simulink model "complex_UIO_alternative_proj_2021_02_16"  (R2019b)
settings: Solver=FixedStepAuto  StartTime=0.0  StopTime=60  FixedStep=0.1  RelTol=1e-3
values from neighbouring files (symbols this model uses):
  Ac = [real(A) -imag(A);imag(A) real(A)]    [DAC_UIO_Comp.m]    (also in LinearND_QUANTUM_2020_11_14_2.m = [realA -imagA;imagA realA]; UIO_alternative_2021_01_26.m; UIO_alternative_PAPER_2021_02_17.m = Abar(2:3,2:3); UIO_alternative_PAPER_2021_03_01.m = Abar(2:3,2:3))
  Amc = [real(Am) -imag(Am);imag(Am) real(Am)]    [DAC_UIO_Comp.m]    (also in UIO_alternative_2021_01_26.m)
  Bc = [real(B) -imag(B);imag(B) real(B)]    [DAC_UIO_Comp.m]    (also in UIO_alternative_2021_01_26.m; UIO_alternative_PAPER_2021_02_17.m = Bbar(2:3,:); UIO_alternative_PAPER_2021_03_01.m = Bbar(2:3,:))
  C = double(subs(C_sym,{ep},{0.1}))    [DAC_UIO_Comp.m]    (also in UIO_adaptive_example.m = [1 0 0 0 0;0 0 0 1 0; 0 0 0 0 1]; UIO_adaptive_example_2.m = [1 0 0 0;0 1 0 0]; UIO_adaptive_example_EEG_Balas_2ch.m = [1, epsilon]; UIO_adaptive_example_alternative_EEG_ch6.m = ss_c.C)
  Fu = mats    [UIO_adaptive_example_alternative_EEG_ch6.m]    (also in UIO_alternative_2021_01_26.m = [0 1 ;-25 0]; UIO_alternative_PAPER_2021_02_17.m = [0,0,0,0, 0;0 0 1 0 0;0 -25 0 0 0;0 0 0 0 1;0 0 0 -144 0]; UIO_alternative_PAPER_2021_03_01.m = [0 1 0 0;-25 0 0 0;0 0 0 1;0 0 -144 0]; UIO_alternative_PAPER_2021_03_02.m = [0 1 0 0;-25 0 0 0;0 0 0 1;0 0 -144 0])
  g1 = 4+2j    [DAC_UIO_Comp.m]    (also in UIO_adaptive_example_EEG_Balas_2ch.m = 4; UIO_alternative_2021_01_26.m = 2+1j; UIO_alternative_PAPER_2021_02_17.m = 2; UIO_alternative_PAPER_2021_03_01.m = 2)
  g2 = 0    [DAC_UIO_Comp.m]    (also in UIO_adaptive_example_EEG_Balas_2ch.m = -0.3; UIO_alternative_2021_01_26.m; UIO_alternative_PAPER_2021_02_17.m = 1; UIO_alternative_PAPER_2021_03_01.m)
  g3 = 0    [DAC_UIO_Comp.m]    (also in UIO_adaptive_example_EEG_Balas_2ch.m = 0.1; UIO_alternative_2021_01_26.m; UIO_alternative_PAPER_2021_02_17.m = -3; UIO_alternative_PAPER_2021_03_01.m)
  gamma_e = 1    [DAC_UIO_Comp.m]    (also in UIO_adaptive_example_EEG_Balas_2ch.m; UIO_adaptive_example_alternative_EEG_ch6.m = .0001*ones(length(Am),1); UIO_alternative_2021_01_26.m = 0.001; UIO_alternative_PAPER_2021_02_17.m = 0.0001)
  K_u = ones(size(Fu,1),1)    [UIO_adaptive_example_alternative_EEG_ch6.m]    (also in UIO_alternative_2021_01_26.m = [0.215;ku]; UIO_alternative_PAPER_2021_02_17.m = [2;10;-1.6;10]; UIO_alternative_PAPER_2021_03_01.m = -[K_cvx(3:end,:)]; UIO_alternative_PAPER_2021_03_02.m)
  Theta = [real(Theta_cust);imag(Theta_cust)]    [LinearND_QUANTUM_2020_11_14_2.m]    (also in UIO_adaptive_example_alternative_EEG_ch6.m = ones(1,size(Fu,1)); UIO_alternative_2021_01_26.m = [1,1]; UIO_alternative_PAPER_2021_02_17.m = [1,1,1,1,1]; UIO_alternative_PAPER_2021_03_01.m = [1,1,1,1])
settings Model: Creator=Tris  LastModifiedBy=Tris

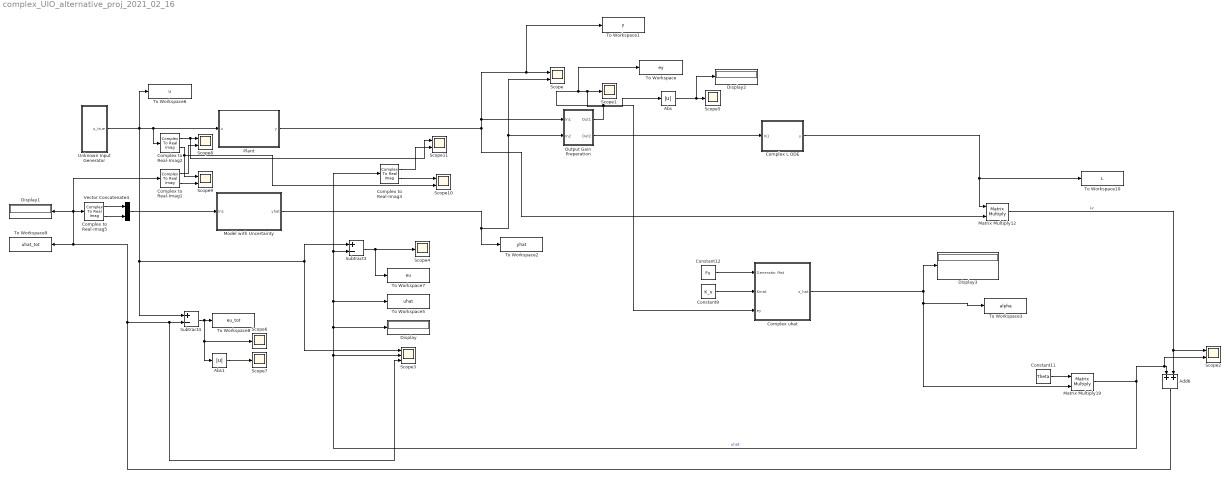
== system complex_UIO_alternative_proj_2021_02_16 ==
  Abs : Abs
  Abs1 : Abs
  Add6 : Sum
  Complex L ODE : Subsystem
  Complex to Real-Imag{1..3,5} (4 alike) : ComplexToRealImag
  "Complex uhat " : Subsystem
  Constant11 : Constant  Value=Theta  VectorParams1D=off
  Constant12 : Constant  Value=Fu
  Constant9 : Constant  Value=K_u  VectorParams1D=off
  Display{,1..3} (4 alike) : Display
  Matrix Multiply12 : Product  Multiplication=Matrix(*)
  Matrix Multiply19 : Product  Multiplication=Matrix(*)
  Model with Uncertainty : Subsystem
  Output Gain Preperation : Subsystem
  Plant : Subsystem
  Scope{,2,8..11} (6 alike) : Scope  NumInputPorts=2
  Scope{1,4..7} (5 alike) : Scope
  Scope3 : Scope  NumInputPorts=3
  Subtract3 : Sum  Inputs=+-
  Subtract4 : Sum  Inputs=+-
  To Workspace : ToWorkspace  VariableName=ey  SaveFormat=Timeseries  SampleTime=-1
  To Workspace1 : ToWorkspace  VariableName=y  SaveFormat=Timeseries  SampleTime=-1
  To Workspace10 : ToWorkspace  VariableName=L  SaveFormat=Timeseries  SampleTime=-1
  To Workspace2 : ToWorkspace  VariableName=yhat  SaveFormat=Timeseries  SampleTime=-1
  To Workspace3 : ToWorkspace  VariableName=alpha  SaveFormat=Timeseries  SampleTime=-1
  To Workspace5 : ToWorkspace  VariableName=uhat  SaveFormat=Timeseries  SampleTime=-1
  To Workspace6 : ToWorkspace  VariableName=u  SaveFormat=Timeseries  SampleTime=-1
  To Workspace7 : ToWorkspace  VariableName=eu  SaveFormat=Timeseries  SampleTime=-1
  To Workspace8 : ToWorkspace  VariableName=eu_tot  SaveFormat=Timeseries  SampleTime=-1
  To Workspace9 : ToWorkspace  VariableName=uhat_tot  SaveFormat=Timeseries  SampleTime=-1
  Unknown Input Generator : Subsystem
  Vector Concatenate4 : Concatenate  Mode=Multidimensional array
  wires:
  Complex to Real-Imag5/2 -> Vector Concatenate4/2
  Complex to Real-Imag5/1 -> Vector Concatenate4/1
  Constant11/1 -> Matrix Multiply19/1
  Matrix Multiply19/1 -> Scope2/2, Add6/1, To Workspace5/1, Complex to Real-Imag3/1, Subtract3/2, Display/1, Scope3/2  "uhat"
  Matrix Multiply12/1 -> Scope2/1, Add6/2  "Ly"
  Add6/1 -> Complex to Real-Imag1/1, Complex to Real-Imag5/1, Display1/1, To Workspace9/1, Scope3/3, Subtract4/2
  Subtract4/1 -> Abs1/1, Scope6/1, To Workspace8/1
  Constant9/1 -> "Complex uhat "/2(Kmat)
  Constant12/1 -> "Complex uhat "/1(Generator Mat)
  "Complex uhat "/1(z_hat) -> To Workspace3/1, Matrix Multiply19/2, Display3/1
  Complex L ODE/1(y) -> To Workspace10/1, Matrix Multiply12/1
  Plant/1(y) -> To Workspace1/1, Scope/1, Output Gain Preperation/1(In1), Matrix Multiply12/2
  Abs/1 -> Display2/1, Scope5/1
  Unknown Input Generator/1(u_true) -> Scope3/1, Subtract3/1, Subtract4/1, To Workspace6/1, Complex to Real-Imag2/1, Plant/1(u)
  Model with Uncertainty/1(yhat) -> To Workspace2/1, Scope/2, Output Gain Preperation/2(In2)
  Vector Concatenate4/1 -> Model with Uncertainty/1(In1)
  Subtract3/1 -> Scope4/1, To Workspace7/1
  Output Gain Preperation/1(Out1) -> To Workspace/1, Abs/1, Scope1/1, "Complex uhat "/3(ey)
  Output Gain Preperation/2(Out2) -> Complex L ODE/1(In1)
  Abs1/1 -> Scope7/1
  Complex to Real-Imag2/1 -> Scope11/1, Scope8/1
  Complex to Real-Imag1/1 -> Scope8/2
  Complex to Real-Imag1/2 -> Scope9/2
  Complex to Real-Imag2/2 -> Scope10/2, Scope9/1
  Complex to Real-Imag3/1 -> Scope11/2
  Complex to Real-Imag3/2 -> Scope10/1

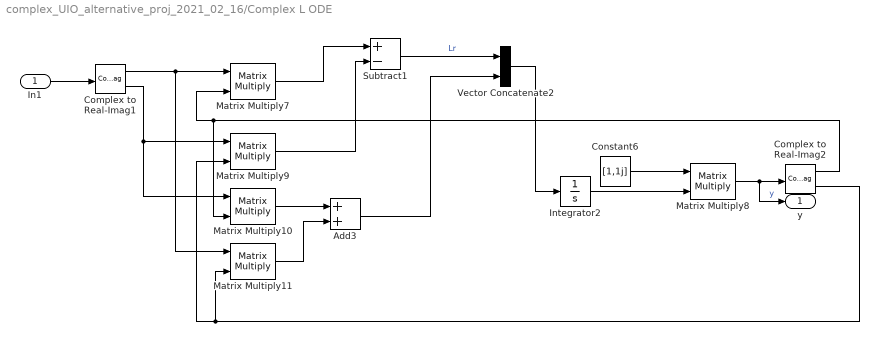
== system complex_UIO_alternative_proj_2021_02_16/Complex L ODE ==
  In1 : Inport
  Add3 : Sum
  Complex to Real-Imag1 : ComplexToRealImag
  Complex to Real-Imag2 : ComplexToRealImag
  Constant6 : Constant  Value=[1,1j]  VectorParams1D=off
  Integrator2 : Integrator  InitialCondition=[1;0.5]
  Matrix Multiply{7..11} (5 alike) : Product  Multiplication=Matrix(*)
  Subtract1 : Sum  Inputs=+-
  Vector Concatenate2 : Concatenate  Mode=Multidimensional array
  y : Outport
  wires:
  Complex to Real-Imag2/1 -> Matrix Multiply7/2, Matrix Multiply10/2
  Matrix Multiply8/1 -> y/1, Complex to Real-Imag2/1  "y"
  Complex to Real-Imag2/2 -> Matrix Multiply11/2, Matrix Multiply9/2
  Subtract1/1 -> Vector Concatenate2/1  "Lr"
  Add3/1 -> Vector Concatenate2/2
  Complex to Real-Imag1/2 -> Matrix Multiply10/1, Matrix Multiply9/1
  Constant6/1 -> Matrix Multiply8/1
  Matrix Multiply10/1 -> Add3/1
  Complex to Real-Imag1/1 -> Matrix Multiply11/1, Matrix Multiply7/1
  Matrix Multiply7/1 -> Subtract1/1
  Integrator2/1 -> Matrix Multiply8/2
  Matrix Multiply9/1 -> Subtract1/2
  Vector Concatenate2/1 -> Integrator2/1
  Matrix Multiply11/1 -> Add3/2
  In1/1 -> Complex to Real-Imag1/1

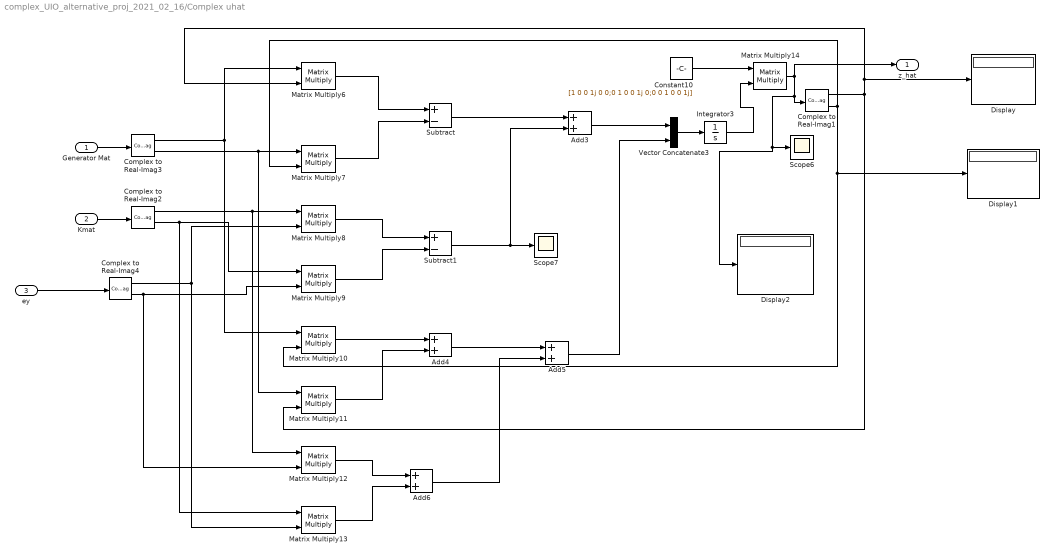
== system complex_UIO_alternative_proj_2021_02_16/Complex uhat  ==
  Generator Mat : Inport
  Kmat : Inport  Port=2
  ey : Inport  Port=3
  Add{3..6} (4 alike) : Sum
  Complex to Real-Imag{1..4} (4 alike) : ComplexToRealImag
  Constant10 : Constant  Value=[1 0 0 1j 0 0;0 1 0 0 1j 0;0 0 1 0 0 1j]  VectorParams1D=off
  Display : Display
  Display1 : Display
  Display2 : Display
  Integrator3 : Integrator  InitialCondition=[2;0;1;0;0;0]  LimitOutput=on
  Matrix Multiply{6..14} (9 alike) : Product  Multiplication=Matrix(*)
  Scope6 : Scope
  Scope7 : Scope
  Subtract : Sum  Inputs=+-
  Subtract1 : Sum  Inputs=+-
  Vector Concatenate3 : Concatenate  Mode=Multidimensional array
  z_hat : Outport
  wires:
  ey/1 -> Complex to Real-Imag4/1
  Matrix Multiply9/1 -> Subtract1/2
  Integrator3/1 -> Matrix Multiply14/2
  Matrix Multiply6/1 -> Subtract/1
  Add5/1 -> Vector Concatenate3/2
  Matrix Multiply14/1 -> Complex to Real-Imag1/1, Scope6/1, Display2/1, z_hat/1
  Matrix Multiply7/1 -> Subtract/2
  Subtract/1 -> Add3/1
  Matrix Multiply13/1 -> Add6/2
  Constant10/1 -> Matrix Multiply14/1
  Add3/1 -> Vector Concatenate3/1
  Vector Concatenate3/1 -> Integrator3/1
  Complex to Real-Imag3/2 -> Matrix Multiply7/1, Matrix Multiply11/1
  Complex to Real-Imag4/1 -> Matrix Multiply13/2, Matrix Multiply8/2
  Generator Mat/1 -> Complex to Real-Imag3/1
  Complex to Real-Imag2/2 -> Matrix Multiply9/1, Matrix Multiply13/1
  Complex to Real-Imag1/2 -> Matrix Multiply7/2, Matrix Multiply10/2, Display1/1
  Add6/1 -> Add5/2
  Add4/1 -> Add5/1
  Complex to Real-Imag4/2 -> Matrix Multiply9/2, Matrix Multiply12/2
  Matrix Multiply10/1 -> Add4/1
  Complex to Real-Imag2/1 -> Matrix Multiply8/1, Matrix Multiply12/1
  Subtract1/1 -> Add3/2, Scope7/1
  Matrix Multiply12/1 -> Add6/1
  Matrix Multiply11/1 -> Add4/2
  Complex to Real-Imag3/1 -> Matrix Multiply10/1, Matrix Multiply6/1
  Kmat/1 -> Complex to Real-Imag2/1
  Complex to Real-Imag1/1 -> Matrix Multiply11/2, Display/1, Matrix Multiply6/2
  Matrix Multiply8/1 -> Subtract1/1

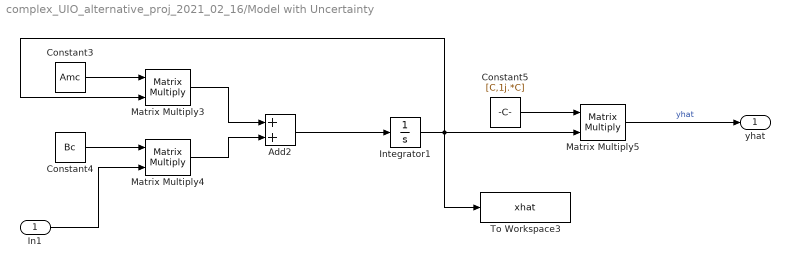
== system complex_UIO_alternative_proj_2021_02_16/Model with Uncertainty ==
  In1 : Inport
  Add2 : Sum
  Constant3 : Constant  Value=Amc
  Constant4 : Constant  Value=Bc  VectorParams1D=off
  Constant5 : Constant  Value=[C,1j.*C]  VectorParams1D=off
  Integrator1 : Integrator
  Matrix Multiply3 : Product  Multiplication=Matrix(*)
  Matrix Multiply4 : Product  Multiplication=Matrix(*)
  Matrix Multiply5 : Product  Multiplication=Matrix(*)
  To Workspace3 : ToWorkspace  VariableName=xhat  SaveFormat=Timeseries  SampleTime=-1
  yhat : Outport
  wires:
  Constant3/1 -> Matrix Multiply3/1
  Integrator1/1 -> To Workspace3/1, Matrix Multiply5/2, Matrix Multiply3/2
  Constant5/1 -> Matrix Multiply5/1
  Add2/1 -> Integrator1/1
  Matrix Multiply4/1 -> Add2/2
  In1/1 -> Matrix Multiply4/2
  Constant4/1 -> Matrix Multiply4/1
  Matrix Multiply3/1 -> Add2/1
  Matrix Multiply5/1 -> yhat/1  "yhat"

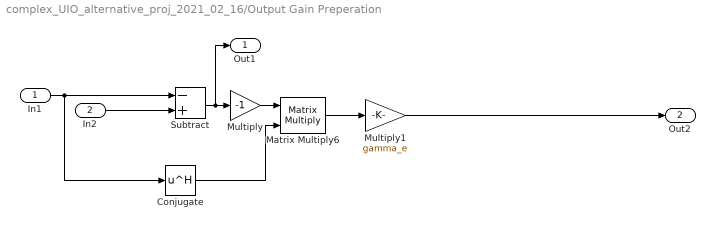
== system complex_UIO_alternative_proj_2021_02_16/Output Gain Preperation ==
  In1 : Inport
  In2 : Inport  Port=2
  Conjugate : Math  Operator=hermitian  RndMeth=Zero  SaturateOnIntegerOverflow=on
  Matrix Multiply6 : Product  Multiplication=Matrix(*)
  Multiply : Gain  Gain=-1
  Multiply1 : Gain  Gain=gamma_e
  Subtract : Sum  Inputs=-+
  Out1 : Outport
  Out2 : Outport  Port=2
  wires:
  Matrix Multiply6/1 -> Multiply1/1
  Multiply1/1 -> Out2/1
  Multiply/1 -> Matrix Multiply6/1
  Conjugate/1 -> Matrix Multiply6/2
  In1/1 -> Conjugate/1, Subtract/1
  In2/1 -> Subtract/2
  Subtract/1 -> Multiply/1, Out1/1

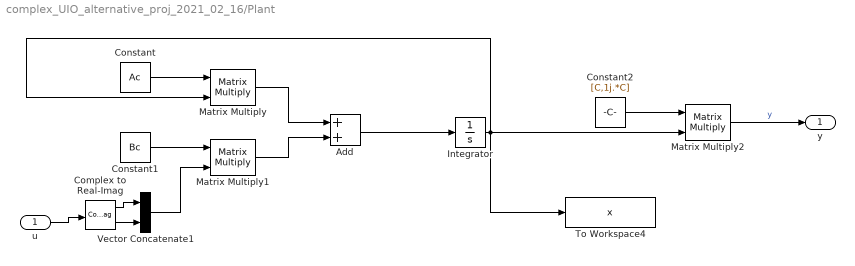
== system complex_UIO_alternative_proj_2021_02_16/Plant ==
  u : Inport
  Add : Sum
  Complex to Real-Imag : ComplexToRealImag
  Constant : Constant  Value=Ac
  Constant1 : Constant  Value=Bc  VectorParams1D=off
  Constant2 : Constant  Value=[C,1j.*C]  VectorParams1D=off
  Integrator : Integrator
  Matrix Multiply : Product  Multiplication=Matrix(*)
  Matrix Multiply1 : Product  Multiplication=Matrix(*)
  Matrix Multiply2 : Product  Multiplication=Matrix(*)
  To Workspace4 : ToWorkspace  VariableName=x  SaveFormat=Timeseries  SampleTime=-1
  Vector Concatenate1 : Concatenate  Mode=Multidimensional array
  y : Outport
  wires:
  Constant2/1 -> Matrix Multiply2/1
  Add/1 -> Integrator/1
  Complex to Real-Imag/1 -> Vector Concatenate1/1
  Constant1/1 -> Matrix Multiply1/1
  u/1 -> Complex to Real-Imag/1
  Matrix Multiply1/1 -> Add/2
  Complex to Real-Imag/2 -> Vector Concatenate1/2
  Integrator/1 -> Matrix Multiply/2, To Workspace4/1, Matrix Multiply2/2
  Constant/1 -> Matrix Multiply/1
  Vector Concatenate1/1 -> Matrix Multiply1/2
  Matrix Multiply/1 -> Add/1
  Matrix Multiply2/1 -> y/1  "y"

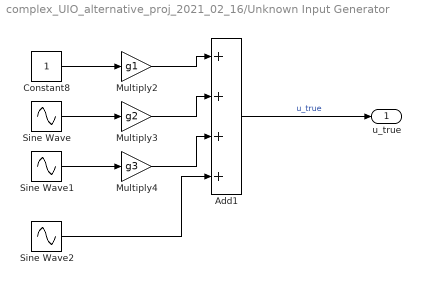
== system complex_UIO_alternative_proj_2021_02_16/Unknown Input Generator ==
  Add1 : Sum  Inputs=++++
  Constant8 : Constant  VectorParams1D=off
  Multiply2 : Gain  Gain=g1
  Multiply3 : Gain  Gain=g2
  Multiply4 : Gain  Gain=g3
  Sine Wave : Sin  Frequency=5  SampleTime=0  VectorParams1D=off
  Sine Wave1 : Sin  Frequency=5  Phase=pi/2  SampleTime=0  VectorParams1D=off
  Sine Wave2 : Sin  Frequency=8  SampleTime=0  VectorParams1D=off
  u_true : Outport
  wires:
  Multiply2/1 -> Add1/1
  Sine Wave1/1 -> Multiply4/1
  Sine Wave/1 -> Multiply3/1
  Multiply4/1 -> Add1/3
  Add1/1 -> u_true/1  "u_true"
  Multiply3/1 -> Add1/2
  Constant8/1 -> Multiply2/1
  Sine Wave2/1 -> Add1/4
